simulink model "ej4_adc_demo"  (Simulink 8.3)
settings: Solver=VariableStepDiscrete  StartTime=0.0  StopTime=1  RelTol=1e-3
libraries: simulink_extras x1
settings Model: Creator=rcheng  LastModifiedBy=Administrador
settings OptimizationCC: ExpressionDepthLimit=2147483647  InitFltsAndDblsToZero=on
settings DebuggingCC: FrameProcessingCompatibilityMsg=error
settings ConfigComp: CovMetricSettings=dw  CovHtmlReporting=on  CovSaveCumulativeToWorkspaceVar=on  CovSaveSingleToWorkspaceVar=on  CovExternalEMLEnable=off  CovSFcnEnable=off

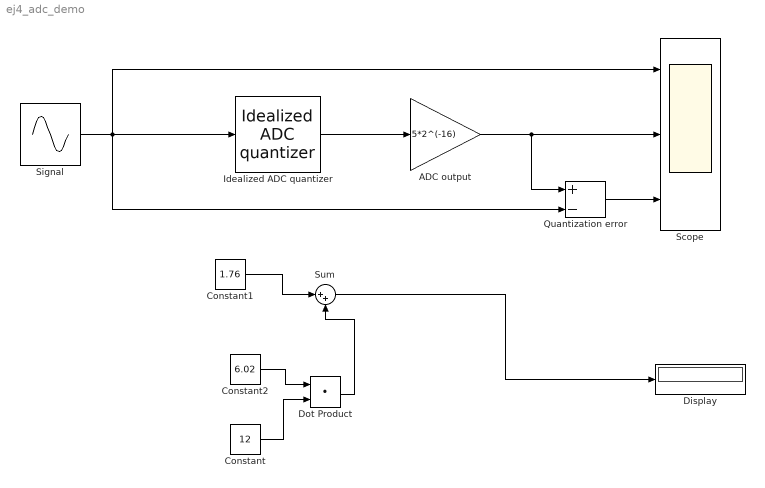
== system ej4_adc_demo ==
  ADC output : Gain  Gain=5*2^(-16)
  Constant : Constant  Value=12
  Constant1 : Constant  Value=1.76
  Constant2 : Constant  Value=6.02
  Display : Display
  Dot Product : DotProduct  InputSameDT=on  OutDataTypeStr=Inherit: Inherit via internal rule
  Idealized ADC quantizer : simulink_extras/Additional Discrete/Idealized ADC quantizer  NumberOfConverterBits=16  Vmin=0  Vmax=5  OutputDataType=uint16  OutputNegativeValues=on
  Quantization error : Sum  Inputs=+-
  Scope : Scope  NumInputPorts=3
      settings: YMin=-5~-5~-5  YMax=5~5~5
  Signal : Sin  Amplitude=2.5  Bias=2.5  Frequency=2*pi*100  SampleTime=1/10000
  Sum : Sum  Inputs=|++
  wires:
  Quantization error/1 -> Scope/3
  Idealized ADC quantizer/1 -> ADC output/1
  ADC output/1 -> Quantization error/1, Scope/2
  Signal/1 -> Idealized ADC quantizer/1, Scope/1, Quantization error/2
  Constant1/1 -> Sum/1
  Constant2/1 -> Dot Product/1
  Constant/1 -> Dot Product/2
  Dot Product/1 -> Sum/2
  Sum/1 -> Display/1
